simulink model "Project1_Option2_Combined"  (R2024b)
settings: Solver=ode4  StartTime=0.0  StopTime=25  FixedStep=1  RelTol=1e-3
values from neighbouring files (symbols this model uses):
  b1 = 1    [Part2_Option1_Code.m]    (also in Part2_Option3_Code.m; Part2_option2_code.m)
  b2 = 1    [Part2_Option1_Code.m]    (also in Part2_Option3_Code.m; Part2_option2_code.m)
  J1 = 100    [Part2_Option1_Code.m]    (also in Part2_Option3_Code.m; Part2_option2_code.m; Project1_Part1_Code_revision_1.m = [100, 0.01]; Project1_Part1_Code_revision_current.m = [100, 0.01])
  J2 = 1    [Part2_Option1_Code.m]    (also in Part2_Option3_Code.m; Part2_option2_code.m)
  omega_init = [10,0]    [Part2_Option1_Code.m]    (also in Part2_Option3_Code.m; Part2_option2_code.m; Project1_Part1_Code_revision_1.m; Project1_Part1_Code_revision_current.m)
  tau = [0, 100]    [Part2_option2_code.m]    (also in Project1_Part1_Code_revision_1.m; Project1_Part1_Code_revision_current.m)
  theta0 = 0    [P1.m]    (also in Part2_Option1_Code.m; Part2_Option3_Code.m; Part2_option2_code.m; Project1_Part1_Code_revision_1.m)
  torque_mode = [1,0]    [P1.m]    (also in Part2_Option1_Code.m = [0,1]; Part2_Option3_Code.m = [0,1]; Part2_option2_code.m = [0,1]; Project1_Part1_Code_revision_1.m = [0,1])
  w_freq = [0.1, 100]    [Part2_Option1_Code.m]    (also in Part2_Option3_Code.m; Part2_option2_code.m; Project1_Part1_Code_revision_current.m)
settings Model: Creator=jacobcody  LastModifiedBy=jacobcody

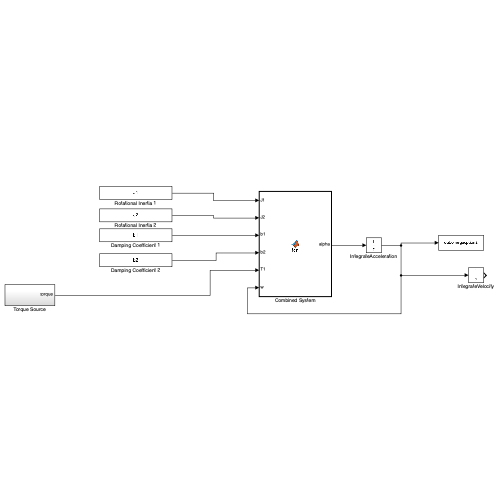
[thumbnail: Simulink's stored preview of the top-level diagram]
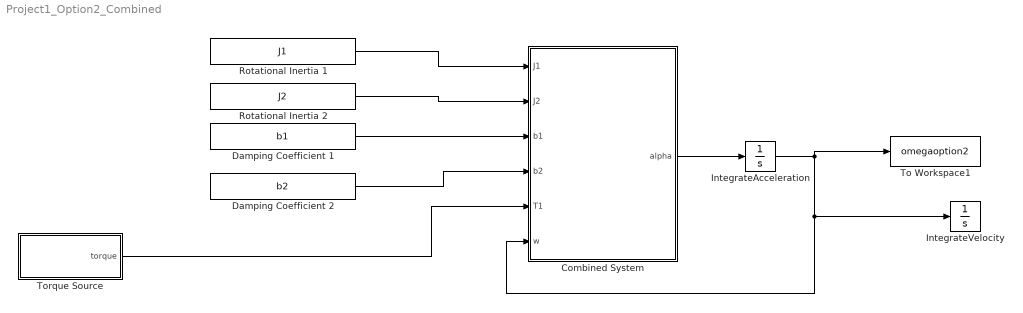
== system Project1_Option2_Combined ==
  Combined System : MATLAB Function  TreatAsAtomicUnit=on
  Damping Coefficient 1 : Constant  Value=b1
  Damping Coefficient 2 : Constant  Value=b2
  IntegrateAcceleration : Integrator  InitialCondition=omega_init
  IntegrateVelocity : Integrator  InitialCondition=theta0
  Rotational Inertia 1 : Constant  Value=J1
  Rotational Inertia 2 : Constant  Value=J2
  To Workspace1 : ToWorkspace  VariableName=omegaoption2  SaveFormat=Timeseries  SampleTime=-1
  Torque Source : Subsystem
  wires:
  Rotational Inertia 1/1 -> Combined System/1(J1)
  IntegrateAcceleration/1 -> To Workspace1/1, IntegrateVelocity/1, Combined System/6(w)
  Torque Source/1(torque) -> Combined System/5(T1)
  Damping Coefficient 1/1 -> Combined System/3(b1)
  Damping Coefficient 2/1 -> Combined System/4(b2)
  Rotational Inertia 2/1 -> Combined System/2(J2)
  Combined System/1(alpha) -> IntegrateAcceleration/1

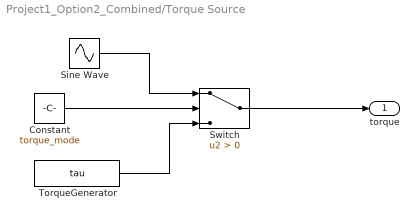
== system Project1_Option2_Combined/Torque Source ==
  Constant : Constant  Value=torque_mode
  Sine Wave : Sin  Frequency=w_freq  SampleTime=0
  Switch : Switch  Criteria=u2 > Threshold  SaturateOnIntegerOverflow=off  InputSameDT=off
  TorqueGenerator : Constant  Value=tau
  torque : Outport
  wires:
  Switch/1 -> torque/1
  Sine Wave/1 -> Switch/1
  TorqueGenerator/1 -> Switch/3
  Constant/1 -> Switch/2

== matlab function Project1_Option2_Combined/Combined System ==
  data: J1 input; J2 input; b1 input; b2 input; T1 input; w input; alpha output
function alpha = fcn(J1, J2, b1, b2, T1, w)
alpha = (1/(J1+J2))*T1-(((b1+b2)/(J1+J2))*w);
